simulink model "smo"  (R2023a)
settings: Solver=VariableStepAuto  StartTime=0.0  StopTime=10.0  RelTol=1e-3
values from neighbouring files (symbols this model uses):
  m = m + 1    (= 2)    [TMO5liubimov.m]    (also in laba2.m = 14; laba3.m = 200; test.m = 5)
  n = 31    [laba2.m]    (also in test.m = 7)
settings Model: Creator=Evangelina  LastModifiedBy=PC
settings RTWCC: GPUComputeCapability=5.0

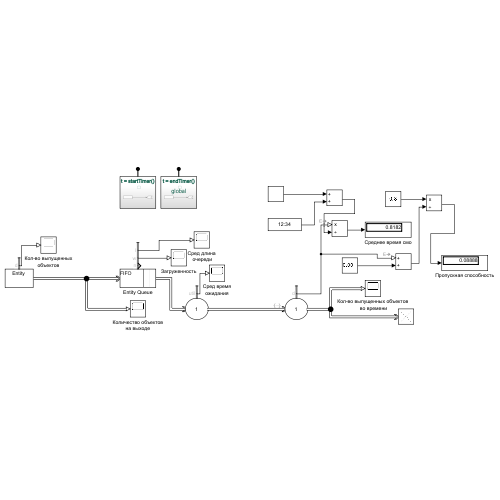
[thumbnail: Simulink's stored preview of the top-level diagram]
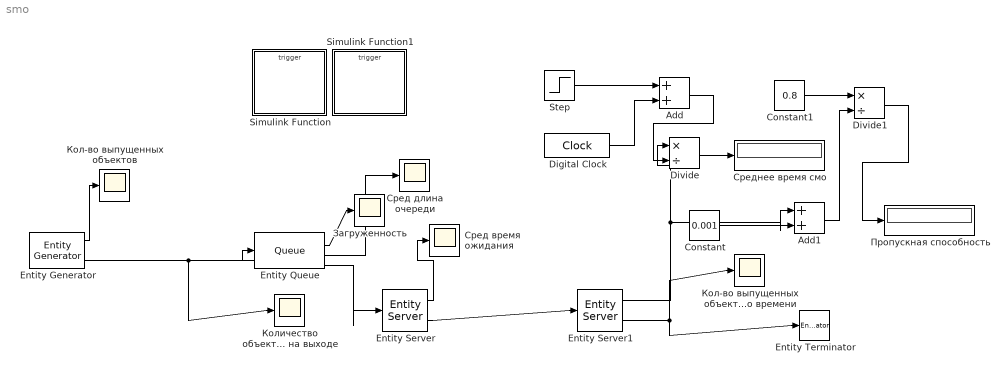
== system smo ==
  Add : Sum
  Add1 : Sum
  Constant : Constant  Value=0.001
  Constant1 : Constant  Value=0.8
  Digital Clock : DigitalClock
  Divide : Product  Inputs=*/
  Divide1 : Product  Inputs=*/
  Entity Generator : EntityGenerator  OutputPortMessageModes=n,m  TimeSource=MATLAB action  IntergenerationTimeAction=|  AttributeName=SMOTime  AttributeInitialValue=0  NumberEntitiesDeparted=on  EntityType=Structured  EntityTypeName=Entity
      | dt = rand(1,1);
      | persistent rngInit;
      | if isempty(rngInit)
      |     seed = 12345;
      |     rng(seed);
      |     rngInit = true;
      | end
      | 
      | mu = 1;
      | x = -mu * log(1 - rand());
      settings: OutputPortMap=o0,o3
  Entity Queue : Queue  InputPortMessageModes=m  OutputPortMessageModes=n,n,n,m  NumberEntitiesInBlock=on  AverageWait=on  AverageQueueLength=on
      settings: OutputPortMap=o1,o2,o3,o5
  Entity Server : EntityServer  InputPortMessageModes=m  OutputPortMessageModes=n,m  Capacity=1  Utilization=on
      settings: OutputPortMap=o5,o9
  Entity Server1 : EntityServer  InputPortMessageModes=m  OutputPortMessageModes=n,m  Capacity=1  ServiceTimeSource=MATLAB action  EntryAction=entity.SMOTime = startTimer();  NumberEntitiesDeparted=on
      settings: OutputPortMap=o0,o9
  Entity Terminator : EntityTerminator  InputPortMessageModes=m
  Simulink Function : Subsystem  TreatAsAtomicUnit=on
  Simulink Function1 : Subsystem  TreatAsAtomicUnit=on
  Step : Step  SampleTime=0
  Загруженность : Scope
  Кол-во выпущенных объектов : Scope
  Кол-во выпущенных объектов во времени : Scope
  Количество объектов на выходе : Scope
  Пропускная способность : Display
  Сред время ожидания : Scope
  Сред длина очереди : Scope
  Среднее время смо : Display
  wires:
  Entity Generator/2 -> Количество объектов на выходе/1, Entity Queue/1
  Entity Generator/1 -> Кол-во выпущенных объектов/1
  Entity Queue/4 -> Entity Server/1
  Entity Server/2 -> Entity Server1/1
  Entity Server1/2 -> Entity Terminator/1, Кол-во выпущенных объектов во времени/1
  Step/1 -> Add/1
  Digital Clock/1 -> Add/2
  Add/1 -> Divide/2
  Entity Server1/1 -> Add1/1, Divide/1
  Divide/1 -> Среднее время смо/1
  Constant/1 -> Add1/2
  Add1/1 -> Divide1/2
  Divide1/1 -> Пропускная способность/1
  Constant1/1 -> Divide1/1
  Entity Queue/3 -> Сред длина очереди/1
  Entity Queue/2 -> Загруженность/1
  Entity Server/1 -> Сред время ожидания/1

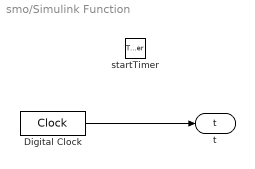
== system smo/Simulink Function ==
  startTimer : TriggerPort  TriggerType=function-call  IsSimulinkFunction=on  FunctionName=startTimer  FunctionVisibility=scoped  VariantControl=(inherit)
  Digital Clock : DigitalClock  SampleTime=-1
  t : ArgOut  DisableCoverage=on  ArgumentName=t
  wires:
  Digital Clock/1 -> t/1

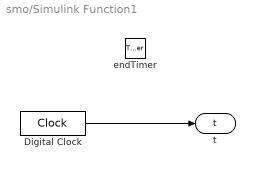
== system smo/Simulink Function1 ==
  endTimer : TriggerPort  TriggerType=function-call  IsSimulinkFunction=on  FunctionName=endTimer  VariantControl=(inherit)
  Digital Clock : DigitalClock  SampleTime=-1
  t : ArgOut  DisableCoverage=on  ArgumentName=t
  wires:
  Digital Clock/1 -> t/1
